simulink model "PrelabSystem"  (R2023a)
settings: Solver=ode45  StartTime=0.0  StopTime=1  RelTol=1e-3
values from neighbouring files (symbols this model uses):
  K = 97/5    (= 19.4)    [Parameters.m]
  Kr = 1+0.6/K    (= 1.03092783505)    [Parameters.m]
settings Model: Creator=Jiadong_Hong  LastModifiedBy=Jiadong_Hong

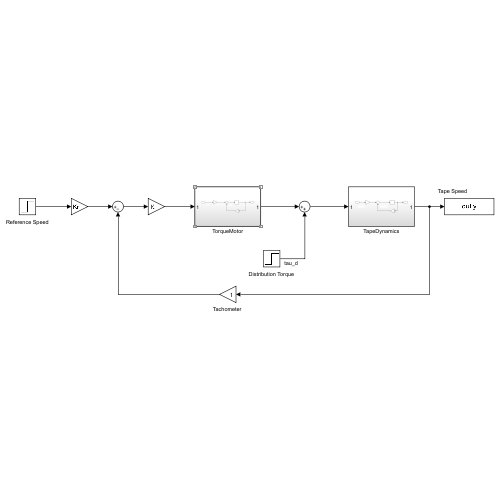
[thumbnail: Simulink's stored preview of the top-level diagram]
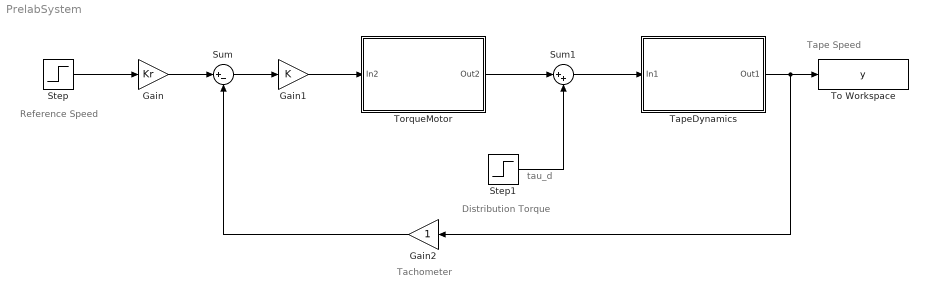
== system PrelabSystem ==
  note: Tachometer
  note: Tape Speed
  note: Reference Speed
  note: Distribution Torque
  note: tau_d
  Gain : Gain  Gain=Kr
  Gain1 : Gain  Gain=K
  Gain2 : Gain
  Step : Step  SampleTime=0
  Step1 : Step  SampleTime=0
  Sum : Sum  Inputs=|+-
  Sum1 : Sum  Inputs=|++
  TapeDynamics : Subsystem
  To Workspace : ToWorkspace  VariableName=y  SampleTime=-1
  TorqueMotor : Subsystem
  wires:
  Step/1 -> Gain/1
  Gain/1 -> Sum/1
  Sum/1 -> Gain1/1
  Gain1/1 -> TorqueMotor/1(In2)
  Step1/1 -> Sum1/2
  TorqueMotor/1(Out2) -> Sum1/1
  Sum1/1 -> TapeDynamics/1(In1)
  TapeDynamics/1(Out1) -> To Workspace/1, Gain2/1
  Gain2/1 -> Sum/2

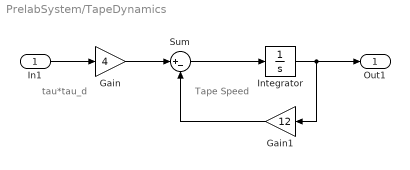
== system PrelabSystem/TapeDynamics ==
  note: tau*tau_d
  note: Tape Speed
  In1 : Inport
  Gain : Gain  Gain=4
  Gain1 : Gain  Gain=12
  Integrator : Integrator
  Sum : Sum  Inputs=|+-
  Out1 : Outport
  wires:
  Integrator/1 -> Gain1/1, Out1/1
  In1/1 -> Gain/1
  Gain1/1 -> Sum/2
  Gain/1 -> Sum/1
  Sum/1 -> Integrator/1

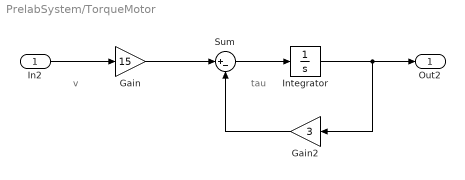
== system PrelabSystem/TorqueMotor ==
  note: v
  note: tau
  In2 : Inport
  Gain : Gain  Gain=15
  Gain2 : Gain  Gain=3
  Integrator : Integrator
  Sum : Sum  Inputs=|+-
  Out2 : Outport
  wires:
  Integrator/1 -> Out2/1, Gain2/1
  Gain2/1 -> Sum/2
  Sum/1 -> Integrator/1
  In2/1 -> Gain/1
  Gain/1 -> Sum/1
